simulink model "s_hover1"  (Simulink 8.8)
settings: Solver=ode1  StartTime=0.0  StopTime=20  FixedStep=0.005  RelTol=1e-3  EnableMultiTasking=on
values from neighbouring files (symbols this model uses):
  CMD_RATE_LIMIT = 60 * pi/180    (= 1.0471975512)    [Copy_of_setup_lab_hover.m]    (also in setup_lab_hover.m; setup_lab_hover1.m)
  K = lqr( A, B, Q, R )    [setup_lab_hover.m]    (also in setup_lab_hover1.m)
  K_AMP = 3    [Copy_of_setup_lab_hover.m]    (also in setup_lab_hover.m; setup_lab_hover1.m)
  V_bias = 2.0    (= 2)    [setup_lab_hover.m]    (also in setup_lab_hover1.m)
  VMAX_AMP = 24    [Copy_of_setup_lab_hover.m]    (also in setup_lab_hover.m; setup_lab_hover1.m)
  VMAX_DAC = 10    [Copy_of_setup_lab_hover.m]    (also in setup_lab_hover.m; setup_lab_hover1.m)
  wcf = 2 * pi * 20    (= 125.663706144)    [Copy_of_setup_lab_hover.m]    (also in setup_lab_hover.m; setup_lab_hover1.m)
  zetaf = 0.6    [Copy_of_setup_lab_hover.m]    (also in setup_lab_hover.m; setup_lab_hover1.m)
undefined symbols (not defined in the file or in its folder): A, B, C, D
libraries: simulink_extras x3, instrumentlib x2, aerolibanimutils x1, simulink x1
settings Model: SuppressorTable=22 serialization::archive 11 0 3 0 0 0 0 0  Creator=hpineros  LastModifiedBy=ronan  ExtModeTrigDuration=10000
settings SolverCC: PositivePriorityOrder=on
settings OptimizationCC: ExpressionDepthLimit=2147483647  InitFltsAndDblsToZero=on
settings DebuggingCC: SaveWithParameterizedLinksMsg=none  SolverPrmCheckMsg=warning
settings RTWCC: SystemTargetFile=quarc_windows.tlc  TemplateMakefile=quarc_default_tmf  Description=QuaRC Win32 Target
settings STFCustomTargetCC: TargetFcnLib=ansi_tfl_tmw.mat  TargetPreCompLibLocation=C:\PROGRA~3\QUARC\lib\2012b\windows\release  GeneratePreprocessorConditionals=Disable all  CPPClassGenCompliant=on  SystemTargetFile=quarc_windows.tlc
settings GRTTargetCC: TargetFcnLib=ansi_tfl_tmw.mat  TargetPreCompLibLocation=C:\PROGRA~3\QUARC\lib\2012b\windows\release  ParMdlRefBuildCompliant=off  CompOptLevelCompliant=off  ConcurrentExecutionCompliant=off  MatFileLogging=off  UseToolchainInfoCompliant=off  ExtMode=on  ExtModeMexFile=quarc_comm

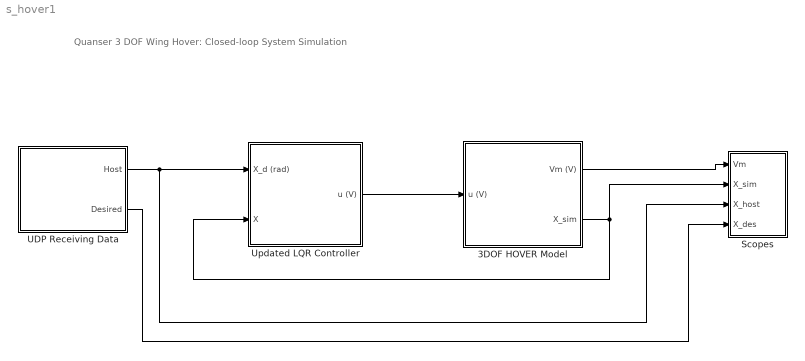
== system s_hover1 ==
  note: Quanser 3 DOF Wing Hover:
      | Closed-loop System Simulation
  3DOF HOVER Model : Subsystem
  Scopes : Subsystem
  "UDP Receiving Data " : Subsystem
  Updated LQR Controller : Subsystem
  wires:
  3DOF HOVER Model/1(Vm (V)) -> Scopes/1(Vm)
  "UDP Receiving Data "/1("Host ") -> Scopes/3(X_host), Updated LQR Controller/1(X_d (rad))
  "UDP Receiving Data "/2("Desired ") -> Scopes/4(X_des)
  Updated LQR Controller/1(u (V)) -> 3DOF HOVER Model/1(u (V))
  3DOF HOVER Model/2(X_sim) -> Updated LQR Controller/2(X), Scopes/2(X_sim)

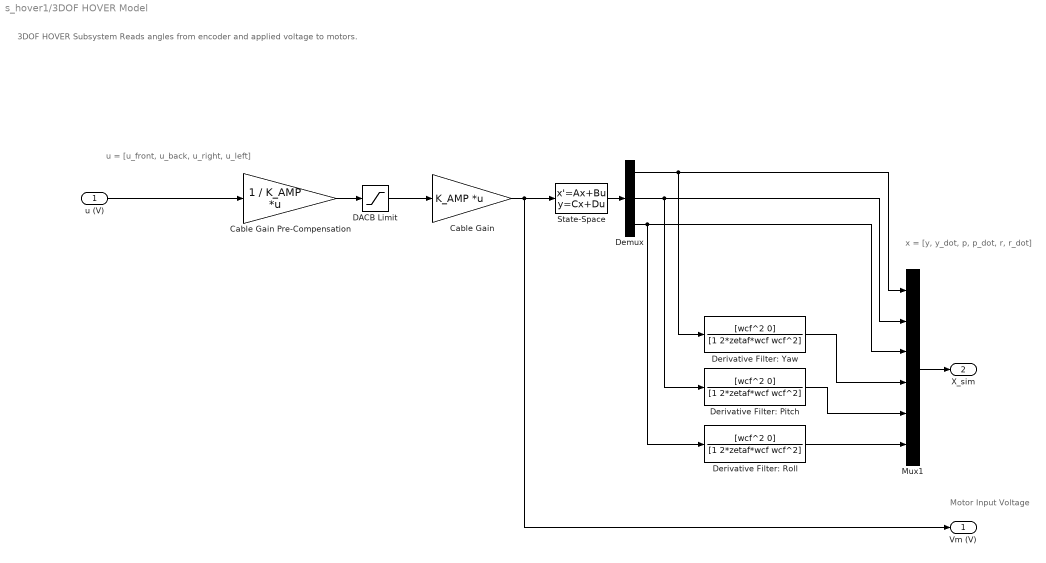
== system s_hover1/3DOF HOVER Model ==
  note: 3DOF HOVER Subsystem
      | Reads angles from encoder and applied voltage to motors.
  note: Motor Input Voltage
  note: u = [u_front, u_back, u_right, u_left]
  note: x = [y, y_dot, p, p_dot, r, r_dot]
  u (V) : Inport
  Cable Gain : Gain  Gain=K_AMP  Multiplication=Matrix(K*u)  SaturateOnIntegerOverflow=on  OutDataTypeStr=Inherit: Same as input  ParamDataTypeStr=Inherit: Same as input
  Cable Gain Pre-Compensation : Gain  Gain=1 / K_AMP  Multiplication=Matrix(K*u)  SaturateOnIntegerOverflow=on  OutDataTypeStr=Inherit: Same as input  ParamDataTypeStr=Inherit: Same as input
  DACB Limit : Saturate  UpperLimit=VMAX_DAC  LowerLimit=-VMAX_DAC
  Demux : Demux  Outputs=3
  Derivative Filter: Pitch : TransferFcn  Numerator=[wcf^2 0]  Denominator=[1 2*zetaf*wcf wcf^2]
  Derivative Filter: Roll : TransferFcn  Numerator=[wcf^2 0]  Denominator=[1 2*zetaf*wcf wcf^2]
  Derivative Filter: Yaw : TransferFcn  Numerator=[wcf^2 0]  Denominator=[1 2*zetaf*wcf wcf^2]
  Mux1 : Mux  Inputs=6
  State-Space : StateSpace  A=A  B=B  C=C  D=D  X0=0
  Vm (V) : Outport
  X_sim : Outport  Port=2
  wires:
  Demux/3 -> Derivative Filter: Roll/1, Mux1/3
  Demux/2 -> Derivative Filter: Pitch/1, Mux1/2
  Derivative Filter: Roll/1 -> Mux1/6
  Derivative Filter: Pitch/1 -> Mux1/5
  Derivative Filter: Yaw/1 -> Mux1/4
  Demux/1 -> Derivative Filter: Yaw/1, Mux1/1
  State-Space/1 -> Demux/1
  Mux1/1 -> X_sim/1
  Cable Gain/1 -> State-Space/1, Vm (V)/1
  DACB Limit/1 -> Cable Gain/1
  Cable Gain Pre-Compensation/1 -> DACB Limit/1
  u (V)/1 -> Cable Gain Pre-Compensation/1

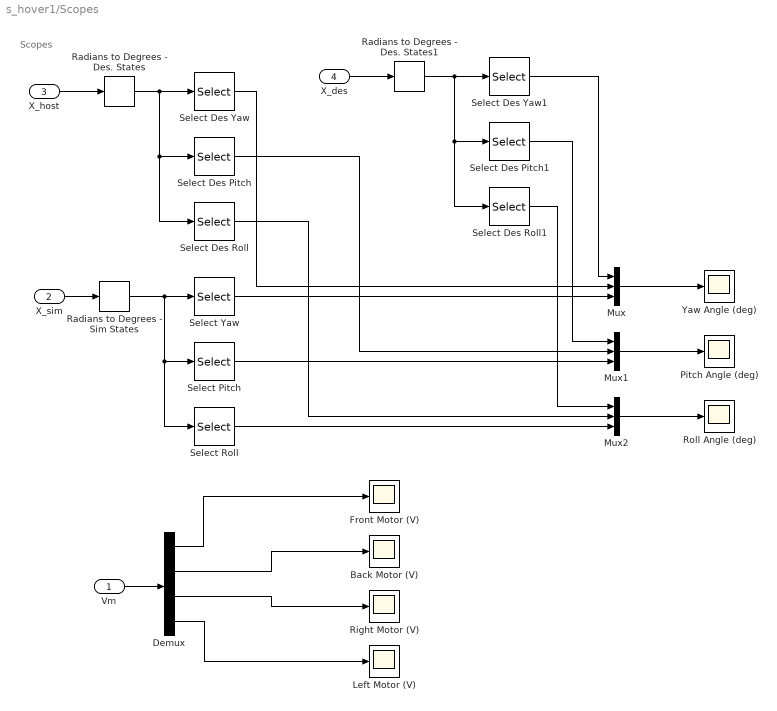
== system s_hover1/Scopes ==
  note: Scopes
  Vm : Inport
  X_sim : Inport  Port=2
  X_host : Inport  Port=3
  X_des : Inport  Port=4
  Back Motor (V) : Scope
  Demux : Demux
  Front Motor (V) : Scope
  Left Motor (V) : Scope
  Mux : Mux  Inputs=3
  Mux1 : Mux  Inputs=3
  Mux2 : Mux  Inputs=3
  Pitch Angle (deg) : Scope
  Radians to Degrees - Des. States : simulink_extras/Transformations/Radians to Degrees
  Radians to Degrees - Des. States1 : simulink_extras/Transformations/Radians to Degrees
  Radians to Degrees - Sim States : simulink_extras/Transformations/Radians to Degrees
  Right Motor (V) : Scope
  Roll Angle (deg) : Scope
  Select Des Pitch : Selector  InputPortWidth=6  IndexOptions=Index vector (dialog)  Indices=2  OutputSizes=1
  Select Des Pitch1 : Selector  InputPortWidth=6  IndexOptions=Index vector (dialog)  Indices=2  OutputSizes=1
  Select Des Roll : Selector  InputPortWidth=6  IndexOptions=Index vector (dialog)  Indices=3  OutputSizes=1
  Select Des Roll1 : Selector  InputPortWidth=6  IndexOptions=Index vector (dialog)  Indices=3  OutputSizes=1
  Select Des Yaw : Selector  InputPortWidth=6  IndexOptions=Index vector (dialog)  Indices=1  OutputSizes=1
  Select Des Yaw1 : Selector  InputPortWidth=6  IndexOptions=Index vector (dialog)  Indices=1  OutputSizes=1
  Select Pitch : Selector  InputPortWidth=6  IndexOptions=Index vector (dialog)  Indices=2  OutputSizes=1
  Select Roll : Selector  InputPortWidth=6  IndexOptions=Index vector (dialog)  Indices=3  OutputSizes=1
  Select Yaw : Selector  InputPortWidth=6  IndexOptions=Index vector (dialog)  Indices=1  OutputSizes=1
  Yaw Angle (deg) : Scope
  wires:
  Radians to Degrees - Des. States/1 -> Select Des Roll/1, Select Des Pitch/1, Select Des Yaw/1
  Mux2/1 -> Roll Angle (deg)/1
  Radians to Degrees - Sim States/1 -> Select Roll/1, Select Pitch/1, Select Yaw/1
  Mux1/1 -> Pitch Angle (deg)/1
  Mux/1 -> Yaw Angle (deg)/1
  X_sim/1 -> Radians to Degrees - Sim States/1
  X_host/1 -> Radians to Degrees - Des. States/1
  Vm/1 -> Demux/1
  Demux/1 -> Front Motor (V)/1
  Demux/2 -> Back Motor (V)/1
  Demux/3 -> Right Motor (V)/1
  Demux/4 -> Left Motor (V)/1
  Radians to Degrees - Des. States1/1 -> Select Des Roll1/1, Select Des Pitch1/1, Select Des Yaw1/1
  X_des/1 -> Radians to Degrees - Des. States1/1
  Select Des Yaw1/1 -> Mux/1
  Select Des Yaw/1 -> Mux/2
  Select Yaw/1 -> Mux/3
  Select Des Pitch1/1 -> Mux1/1
  Select Des Pitch/1 -> Mux1/2
  Select Pitch/1 -> Mux1/3
  Select Des Roll/1 -> Mux2/2
  Select Roll/1 -> Mux2/3
  Select Des Roll1/1 -> Mux2/1

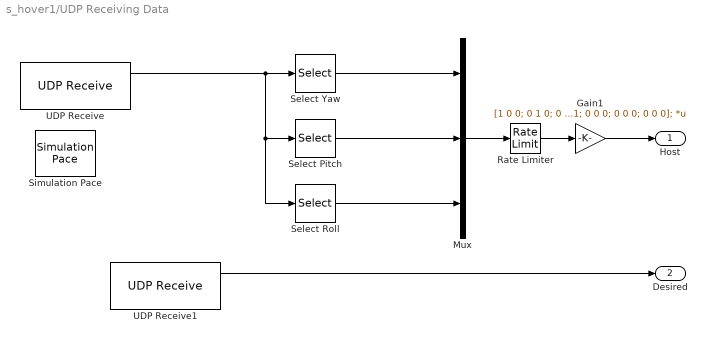
== system s_hover1/UDP Receiving Data  ==
  Gain1 : Gain  Gain=[1 0 0; 0 1 0; 0 0 1; 0 0 0; 0 0 0; 0 0 0];  Multiplication=Matrix(K*u)
  Mux : Mux  Inputs=3
  Rate Limiter : RateLimiter  RisingSlewLimit=CMD_RATE_LIMIT  FallingSlewLimit=-CMD_RATE_LIMIT  SampleTimeMode=inherited
  Select Pitch : Selector  InputPortWidth=6  IndexOptions=Index vector (dialog)  Indices=2  OutputSizes=1
  Select Roll : Selector  InputPortWidth=6  IndexOptions=Index vector (dialog)  Indices=3  OutputSizes=1
  Select Yaw : Selector  InputPortWidth=6  IndexOptions=Index vector (dialog)  Indices=1  OutputSizes=1
  Simulation Pace : aerolibanimutils/Simulation Pace  SimulationPace=1  SleepMode=MATLAB Thread  OutputPaceError=off  SampleTime=0.005
  UDP Receive : instrumentlib/UDP Receive  Host=localhost  Port=9091  LocalPort=9092  DataSize="[6  1]"  EnableBlockingMode=off  Timeout=10  SampleTime=0.005  DataType=double  ByteOrder=BigEndian
  UDP Receive1 : instrumentlib/UDP Receive  Host=localhost  Port=9093  LocalPort=9094  DataSize="[6  1]"  EnableBlockingMode=off  Timeout=10  SampleTime=0.005  DataType=double  ByteOrder=BigEndian
  "Host " : Outport
  "Desired " : Outport  Port=2
  wires:
  Select Roll/1 -> Mux/3
  Select Pitch/1 -> Mux/2
  Select Yaw/1 -> Mux/1
  UDP Receive/1 -> Select Roll/1, Select Pitch/1, Select Yaw/1
  Mux/1 -> Rate Limiter/1
  Rate Limiter/1 -> Gain1/1
  Gain1/1 -> "Host "/1
  UDP Receive1/1 -> "Desired "/1

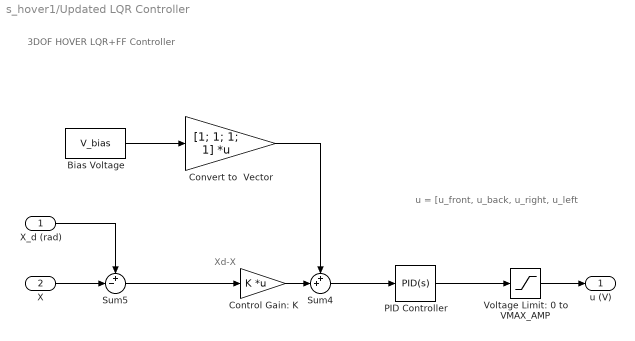
== system s_hover1/Updated LQR Controller ==
  note: u = [u_front, u_back, u_right, u_left
  note: Xd-X
  note: 3DOF HOVER LQR+FF Controller
  X_d (rad) : Inport
  X : Inport  Port=2
  Bias Voltage : Constant  Value=V_bias
  Control Gain: K : Gain  Gain=K  Multiplication=Matrix(K*u)
  Convert to  Vector : Gain  Gain=[1; 1; 1; 1]  Multiplication=Matrix(K*u)
  PID Controller : simulink/Continuous/PID Controller  Controller=PID  TimeDomain=Continuous-time  SampleTime=-1  IntegratorMethod=Forward Euler  FilterMethod=Forward Euler  Form=Parallel  UseFilter=on  ControllerParametersSource=internal  P=2.1  I=0.05  D=0  N=100  InitialConditionSource=internal  InitialConditionForIntegrator=0  InitialConditionForFilter=0  ExternalReset=none  LimitOutput=off  UpperSaturationLimit=inf  LowerSaturationLimit=-inf  LinearizeAsGain=on  AntiWindupMode=none  Kb=1  TrackingMode=off  Kt=1  PParamMin=[]  PParamMax=[]  IParamMin=[]  IParamMax=[]  DParamMin=[]  DParamMax=[]  NParamMin=[]  NParamMax=[]  KbParamMin=[]  KbParamMax=[]  KtParamMin=[]  KtParamMax=[]  POutMin=[]  POutMax=[]  IOutMin=[]  IOutMax=[]  DOutMin=[]  DOutMax=[]  NOutMin=[]  NOutMax=[]  KbOutMin=[]  KbOutMax=[]  KtOutMin=[]  KtOutMax=[]  IntegratorOutMin=[]  IntegratorOutMax=[]  FilterOutMin=[]  FilterOutMax=[]  SumOutMin=[]  SumOutMax=[]  SumI1OutMin=[]  SumI1OutMax=[]  SumI2OutMin=[]  SumI2OutMax=[]  SumI3OutMin=[]  SumI3OutMax=[]  SumDOutMin=[]  SumDOutMax=[]  SaturationOutMin=[]  SaturationOutMax=[]  IntegratorContinuousStateAttributes=''  IntegratorStateMustResolveToSignalObject=off  IntegratorRTWStateStorageClass=Auto  FilterContinuousStateAttributes=''  FilterStateMustResolveToSignalObject=off  FilterRTWStateStorageClass=Auto  DifferentiatorICPrevScaledInput=0  DifferentiatorOutMin=[]  DifferentiatorOutMax=[]
  Sum4 : Sum  Inputs=++|
  Sum5 : Sum  Inputs=+-|
  Voltage Limit: 0 to VMAX_AMP : Saturate  UpperLimit=VMAX_AMP  LowerLimit=0
  u (V) : Outport
  wires:
  X/1 -> Sum5/2
  X_d (rad)/1 -> Sum5/1
  Convert to  Vector/1 -> Sum4/1
  Control Gain: K/1 -> Sum4/2
  Bias Voltage/1 -> Convert to  Vector/1
  Voltage Limit: 0 to VMAX_AMP/1 -> u (V)/1
  Sum5/1 -> Control Gain: K/1
  Sum4/1 -> PID Controller/1
  PID Controller/1 -> Voltage Limit: 0 to VMAX_AMP/1
